simulink model "openloop_control"  (R2023b)
settings: Solver=FixedStepAuto  StartTime=0.0  StopTime=15.0  FixedStep=0.001  RelTol=1e-3
values from neighbouring files (symbols this model uses):
  a = [q1, q2, q3, J]    [observer_for_disturbance_par.m]    (also in openloop_control_par.m; state_feedback_around_eq_par.m)
  a_vect = -At(2,:)'    [openloop_control_par.m]
  alpha_vect = poly3traj(z0,zT,H)    [openloop_control_par.m]
  x0 = [2; 200; 0]    [observer_for_disturbance_par.m]    (also in openloop_control_par.m = [ 2 ; 200 ]; state_feedback_around_eq_par.m = [2; 200])
settings Model: Creator=peterparker  LastModifiedBy=peterparker

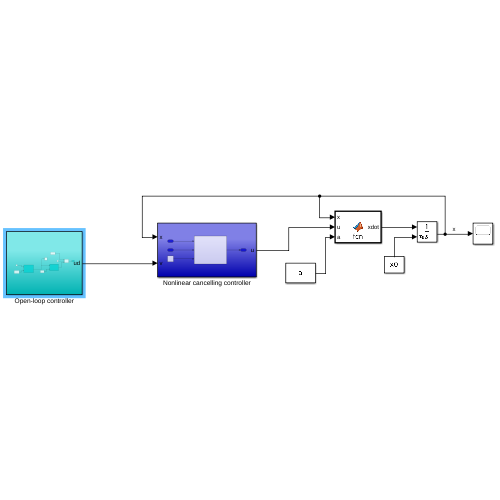
[thumbnail: Simulink's stored preview of the top-level diagram]
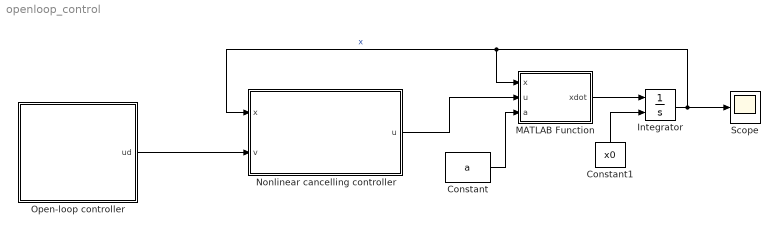
== system openloop_control ==
  Constant : Constant  Value=a
  Constant1 : Constant  Value=x0
  Integrator : Integrator  InitialConditionSource=external
  MATLAB Function : MATLAB Function  TreatAsAtomicUnit=on
  Nonlinear cancelling controller : Subsystem
  Open-loop controller : Subsystem
  Scope : Scope
  wires:
  Constant/1 -> MATLAB Function/3(a)
  MATLAB Function/1(xdot) -> Integrator/1
  Integrator/1 -> Nonlinear cancelling controller/1(x), MATLAB Function/1(x), Scope/1  "x"
  Constant1/1 -> Integrator/2
  Nonlinear cancelling controller/1(u) -> MATLAB Function/2(u)
  Open-loop controller/1(ud) -> Nonlinear cancelling controller/2(v)

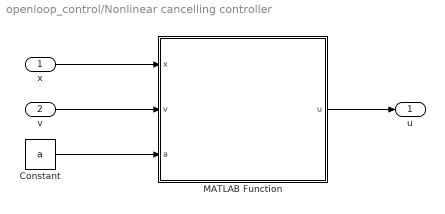
== system openloop_control/Nonlinear cancelling controller ==
  x : Inport
  v : Inport  Port=2
  Constant : Constant  Value=a  VectorParams1D=off
  MATLAB Function : MATLAB Function  TreatAsAtomicUnit=on
  u : Outport
  wires:
  x/1 -> MATLAB Function/1(x)
  v/1 -> MATLAB Function/2(v)
  MATLAB Function/1(u) -> u/1
  Constant/1 -> MATLAB Function/3(a)

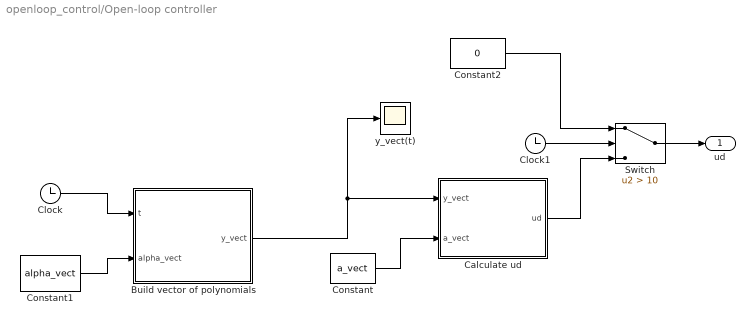
== system openloop_control/Open-loop controller ==
  Build vector of polynomials : MATLAB Function  TreatAsAtomicUnit=on
  Calculate ud : MATLAB Function  TreatAsAtomicUnit=on
  Clock : Clock
  Clock1 : Clock
  Constant : Constant  Value=a_vect  VectorParams1D=off
  Constant1 : Constant  Value=alpha_vect  VectorParams1D=off
  Constant2 : Constant  Value=0
  Switch : Switch  Criteria=u2 > Threshold  Threshold=10  SaturateOnIntegerOverflow=off  InputSameDT=off
  y_vect(t) : Scope
  ud : Outport
  wires:
  Build vector of polynomials/1(y_vect) -> y_vect(t)/1, Calculate ud/1(y_vect)
  Constant/1 -> Calculate ud/2(a_vect)
  Constant1/1 -> Build vector of polynomials/2(alpha_vect)
  Clock/1 -> Build vector of polynomials/1(t)
  Calculate ud/1(ud) -> Switch/3
  Switch/1 -> ud/1
  Clock1/1 -> Switch/2
  Constant2/1 -> Switch/1

== matlab function openloop_control/Open-loop controller/Build vector of polynomials ==
  data: t input; y_vect output; alpha_vect input
function y_vect = fcn(t,alpha_vect)

if length(alpha_vect) == 4
    t_vect0 = [ 1 ; t ; t^2 ; t^3 ]; % vector of t values
    t_vect1 = [ 0 ; 1 ; 2*t ; 3*t^2 ]; % derivative of t_vect0
    t_vect2 = [ 0 ; 0 ; 2 ; 2*3*t ]; % derivative of t_vect1
elseif length(alpha_vect) == 6
    t_vect0 = [ 1 ; t ; t^2 ; t^3 ; t^4 ; t^5 ]; % vector of t values
    t_vect1 = [ 0 ; 1 ; 2*t ; 3*t^2 ; 4*t^3 ; 5*t^4 ]; % derivative of t_vect0
    t_vect2 = [ 0 ; 0 ; 2 ; 2*3*t ; 3*4*t^2 ; 4*5*t^3 ]; % derivative of t_vect1
else 
    t_vect0 = [ 1 ; t ; t^2 ; t^3 ; t^4 ; t^5 ; t^6 ; t^7 ]; % vector of t values
    t_vect1 = [ 0 ; 1 ; 2*t ; 3*t^2 ; 4*t^3 ; 5*t^4 ; 6*t^5 ; 7*t^6 ]; % derivative of t_vect0
    t_vect2 = [ 0 ; 0 ; 2 ; 2*3*t ; 3*4*t^2 ; 4*5*t^3 ; 5*6*t^4 ; 6*7*t^5 ]; % derivative of t_vect1
end


yd = t_vect0'*alpha_vect;
yd_dot = t_vect1'*alpha_vect;
yd_ddot = t_vect2'*alpha_vect;

% vector of desired trajectory and its derivatives
y_vect = [ yd ; yd_dot ; yd_ddot ];

== matlab function openloop_control/MATLAB Function ==
  data: x input; u input; xdot output; a input
function xdot = fcn(x,u, a)

q1 = a(1);
q2 = a(2);
q3 = a(3);
J = a(4);


xdot = [-q1 * x(2) * x(1) + u; 
        q2/J * x(1) - q3/J * x(2)];

== matlab function openloop_control/Open-loop controller/Calculate ud ==
  data: y_vect input; ud output; a_vect input
function ud = fcn(y_vect,a_vect)

a_vect = [ a_vect ; 1 ];


% computation open-loop input
ud = a_vect' * y_vect;

== matlab function openloop_control/Nonlinear cancelling controller/MATLAB Function ==
  data: x input; v input; u output; a input
function u = c_lin(x,v,a)

% a is the vector of constant parameters
q1 = a(1);

% cancelling controller
u = q1*x(1)*x(2) + v;
